simulink model "MOS2_UE04"  (R2022b)
settings: Solver=ode4  StartTime=0.0  StopTime=100  FixedStep=0.01  RelTol=1e-3
undefined symbols (not defined in the file or in its folder): sigbuilder_block
settings Model: Creator=basti  LastModifiedBy=basti
settings DebuggingCC: UnconnectedInputMsg=warning  UnconnectedOutputMsg=warning  UnconnectedLineMsg=warning
settings ModelReferenceCC: EnableRefExpFcnMdlSchedulingChecks=on
settings RTWCC: DLArmComputeVersion=19.05

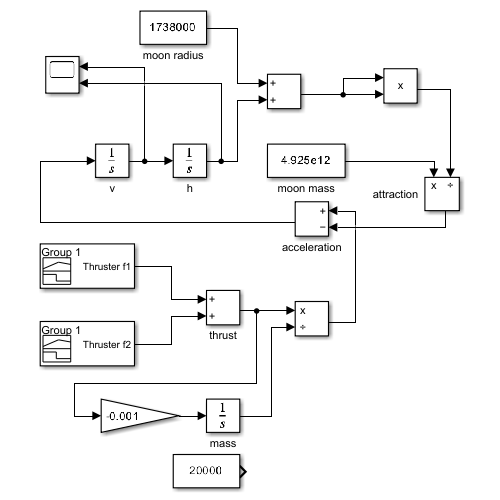
[thumbnail: Simulink's stored preview of the top-level diagram]
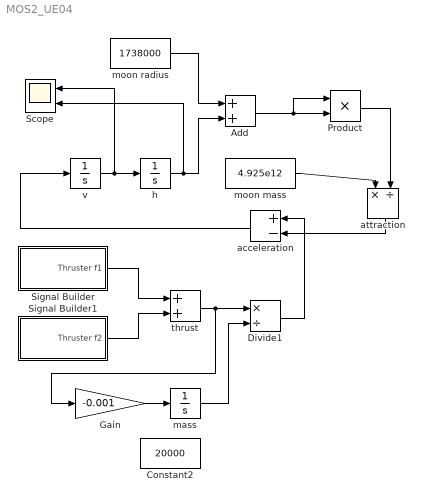
== system MOS2_UE04 ==
  Add : Sum
  Constant2 : Constant  Value=20000
  Divide1 : Product  Inputs=*/
  Gain : Gain  Gain=-0.001
  Product : Product
  Scope : Scope  NumInputPorts=2
  Signal Builder : Subsystem  Tag=STV Subsys  LoadFcn=sigbuilder_block('load');  StartFcn=sigbuilder_block('start');  StopFcn=sigbuilder_block('stop');  ClipboardFcn=sigbuilder_block('clipboard');  mask(Sigbuilder block){tuvar=[0:10]}
      mask help: Simulink:masks:SigbuilderBlock_MD
      mask init:
      | if ~strcmp(get_param(bdroot(gcbh),'SimulationStatus'),'stopped') tuvar = sigbuilder_block('maskInit'); end
      settings: CopyFcn=sigbuilder_block('copy');  DeleteFcn=sigbuilder_block('delete');  ModelCloseFcn=sigbuilder_block('modelClose');  PreSaveFcn=sigbuilder_block('preSave');  PauseFcn=sigbuilder_block('pause');  ContinueFcn=sigbuilder_block('continue');  NameChangeFcn=sigbuilder_block('namechange');  OpenFcn=sigbuilder_block('open',[437.6 199.2 550.4 400 ]);  CloseFcn=sigbuilder_block('close');
      mask Display: plot(0, 0, 100, 100,[2, 2, 32, 32, 2], [68, 8, 8, 68, 68],[32, 2], [38, 38], [32, 19, 2],[53, 60, 44], [32, 17, 17, 2],[16, 16, 31, 31]);txt = getActiveGroup(gcbh);text(2, 100, txt,'verticalAlignment', 'top');
  Signal Builder1 : Subsystem  Tag=STV Subsys  LoadFcn=sigbuilder_block('load');  StartFcn=sigbuilder_block('start');  StopFcn=sigbuilder_block('stop');  ClipboardFcn=sigbuilder_block('clipboard');  mask(Sigbuilder block){tuvar=[0:10]}
      mask help: Simulink:masks:SigbuilderBlock_MD
      mask init:
      | if ~strcmp(get_param(bdroot(gcbh),'SimulationStatus'),'stopped') tuvar = sigbuilder_block('maskInit'); end
      settings: CopyFcn=sigbuilder_block('copy');  DeleteFcn=sigbuilder_block('delete');  ModelCloseFcn=sigbuilder_block('modelClose');  PreSaveFcn=sigbuilder_block('preSave');  PauseFcn=sigbuilder_block('pause');  ContinueFcn=sigbuilder_block('continue');  NameChangeFcn=sigbuilder_block('namechange');  OpenFcn=sigbuilder_block('open',[437.6 186 550.4 400.2 ]);  CloseFcn=sigbuilder_block('close');
      mask Display: plot(0, 0, 100, 100,[2, 2, 32, 32, 2], [68, 8, 8, 68, 68],[32, 2], [38, 38], [32, 19, 2],[53, 60, 44], [32, 17, 17, 2],[16, 16, 31, 31]);txt = getActiveGroup(gcbh);text(2, 100, txt,'verticalAlignment', 'top');
  acceleration : Sum  Inputs=+-
  attraction : Product  Inputs=*/
  h : Integrator  InitialCondition=1000
  mass : Integrator  InitialCondition=20000
  moon mass : Constant  Value=4.925e12
  moon radius : Constant  Value=1738000
  thrust : Sum
  v : Integrator  InitialCondition=-10
  wires:
  v/1 -> Scope/1, h/1
  h/1 -> Scope/2, Add/2
  moon radius/1 -> Add/1
  Add/1 -> Product/1, Product/2
  Signal Builder/1(Thruster f1) -> thrust/1
  Signal Builder1/1(Thruster f2) -> thrust/2
  Product/1 -> attraction/2
  moon mass/1 -> attraction/1
  mass/1 -> Divide1/2
  thrust/1 -> Gain/1, Divide1/1
  Divide1/1 -> acceleration/1
  attraction/1 -> acceleration/2
  acceleration/1 -> v/1
  Gain/1 -> mass/1

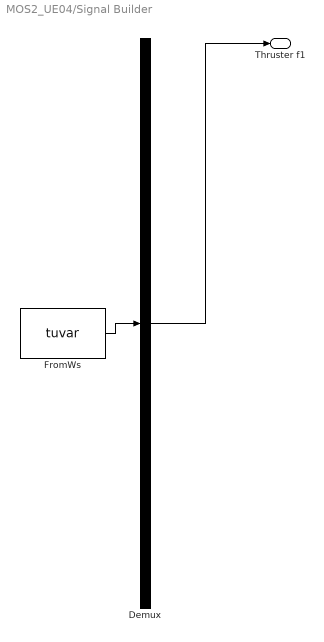
== system MOS2_UE04/Signal Builder ==
  Demux : Demux  Tag=STV Demux  Outputs=1
      settings: DisplayOption=none
  FromWs : FromWorkspace  Tag=STV FromWs  VariableName=tuvar
      SigBuilderData=|
      | common.afterFinalStr = 'Extrapolate'
      | common.sampleTime = 0
      | dataSet.timeRange = [0 100]
      | dataSet.name = 'Group 1'
      | sbobj.Groups.Name = 'Group 1'
      | sbobj.Groups.Signals.Name = 'Thruster f1'
      | sbobj.Groups.Signals.XData = [0 27 27 40 40 100]
      | sbobj.Groups.Signals.YData = [0 0 42000 42000 0 0]
      | sbobj.Groups.TimeRange = [0 100]
  Thruster f1 : Outport  Tag=STV Outport
  wires:
  Demux/1 -> Thruster f1/1
  FromWs/1 -> Demux/1

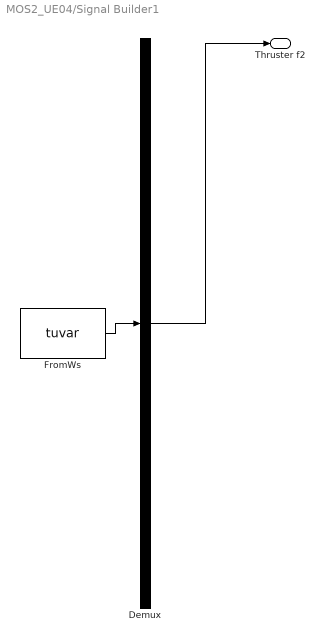
== system MOS2_UE04/Signal Builder1 ==
  Demux : Demux  Tag=STV Demux  Outputs=1
      settings: DisplayOption=none
  FromWs : FromWorkspace  Tag=STV FromWs  VariableName=tuvar
      SigBuilderData=|
      | common.afterFinalStr = 'Extrapolate'
      | common.sampleTime = 0
      | dataSet.timeRange = [0 100]
      | dataSet.name = 'Group 1'
      | sbobj.Groups.Name = 'Group 1'
      | sbobj.Groups.Signals.Name = 'Thruster f2'
      | sbobj.Groups.Signals.XData = [0 15.4 15.4 43 43 100]
      | sbobj.Groups.Signals.YData = [0 0 34000 34000 0 0]
      | sbobj.Groups.TimeRange = [0 100]
  Thruster f2 : Outport  Tag=STV Outport
  wires:
  Demux/1 -> Thruster f2/1
  FromWs/1 -> Demux/1
